simulink model "three_phase_hw_x"  (Simulink 6.1)
settings: Solver=ode23tb  StartTime=0.0  StopTime=0.14999  MaxStep=1e-4  RelTol=1e-3  AbsTol=.01
libraries: powerlib x17
settings Model: LastModifiedBy=ThinkPad
settings DebuggingCC: SolverPrmCheckMsg=warning

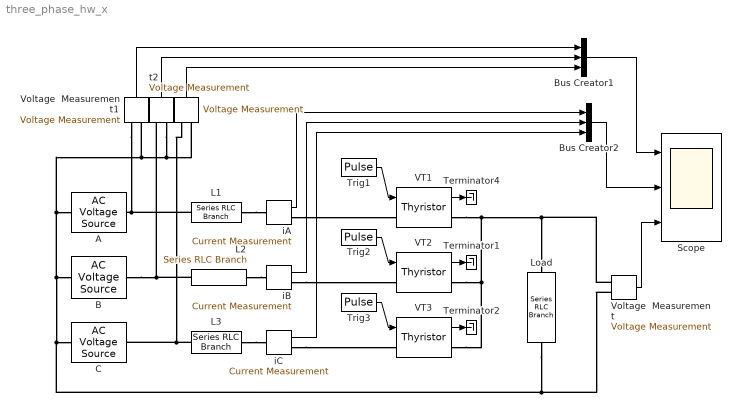
== system three_phase_hw_x ==
  "   " : powerlib/Measurements/Voltage Measurement  Orientation=up  PhasorSimulation=off  OutputType=Complex  PSBequivalent=0
  A : powerlib/Electrical Sources/AC Voltage Source  Amplitude=100  Phase=30  Frequency=50  SampleTime=0  Measurements=None
  B : powerlib/Electrical Sources/AC Voltage Source  Amplitude=100  Phase=-90  Frequency=50  SampleTime=0  Measurements=None
  Bus Creator1 : BusCreator  DialogController=Simulink.DDGSource_Bus  Inputs=3
  Bus Creator2 : BusCreator  DialogController=Simulink.DDGSource_Bus  Inputs=3
  C : powerlib/Electrical Sources/AC Voltage Source  Amplitude=100  Phase=-210  Frequency=50  SampleTime=0  Measurements=None
  L1 : powerlib/Elements/Series RLC Branch  Orientation=left  PhysicalDomain=powersysdomain  SubClassName=unknown  LeftPortType=p1  RightPortType=p1  LConnTagsString=__new0  RConnTagsString=__new0  Resistance=0  Inductance=0.002  Capacitance=inf  Measurements=None
  L2 : powerlib/Elements/Series RLC Branch  Orientation=left  PhysicalDomain=powersysdomain  SubClassName=unknown  LeftPortType=p1  RightPortType=p1  LConnTagsString=__new0  RConnTagsString=__new0  Resistance=0  Inductance=0.002  Capacitance=inf  Measurements=None
  L3 : powerlib/Elements/Series RLC Branch  Orientation=left  PhysicalDomain=powersysdomain  SubClassName=unknown  LeftPortType=p1  RightPortType=p1  LConnTagsString=__new0  RConnTagsString=__new0  Resistance=0  Inductance=0.002  Capacitance=inf  Measurements=None
  Load : powerlib/Elements/Series RLC Branch  Orientation=down  PhysicalDomain=powersysdomain  SubClassName=unknown  LeftPortType=p1  RightPortType=p1  LConnTagsString=__new0  RConnTagsString=__new0  Resistance=2  Inductance=0.05  Capacitance=inf  Measurements=None
  Scope : Scope  NumInputPorts=3
      settings: TimeRange=0.05  YMin=-100~0~-100  YMax=100~50~100  Decimation=5  SampleInput=on  SampleTime=1e-4
  Terminator1 : Terminator
  Terminator2 : Terminator
  Terminator4 : Terminator
  Trig1 : DiscretePulseGenerator  PulseType=Time based  Amplitude=10  Period=0.02  PulseWidth=5  PhaseDelay=0.00167
  Trig2 : DiscretePulseGenerator  PulseType=Time based  Amplitude=10  Period=0.02  PulseWidth=5  PhaseDelay=0.00833
  Trig3 : DiscretePulseGenerator  PulseType=Time based  Amplitude=10  Period=0.02  PulseWidth=5  PhaseDelay=0.015
  VT1 : powerlib/Power Electronics/Thyristor  Ron=0.01  Lon=0  Vf=0.8  IC=0  Rs=1000  Cs=100e-9  Measurements=on
  VT2 : powerlib/Power Electronics/Thyristor  Ron=0.01  Lon=0  Vf=0.8  IC=0  Rs=1000  Cs=100e-9  Measurements=on
  VT3 : powerlib/Power Electronics/Thyristor  Ron=0.01  Lon=0  Vf=0.8  IC=0  Rs=1000  Cs=100e-9  Measurements=on
  Voltage  Measurement : powerlib/Measurements/Voltage Measurement  PhasorSimulation=off  OutputType=Complex  PSBequivalent=0
  Voltage  Measurement1 : powerlib/Measurements/Voltage Measurement  Orientation=up  PhasorSimulation=off  OutputType=Complex  PSBequivalent=0
  iA : powerlib/Measurements/Current Measurement  PhasorSimulation=off  OutputType=Complex  PSBequivalent=0
  iB : powerlib/Measurements/Current Measurement  PhasorSimulation=off  OutputType=Complex  PSBequivalent=0
  iC : powerlib/Measurements/Current Measurement  PhasorSimulation=off  OutputType=Complex  PSBequivalent=0
  t2 : powerlib/Measurements/Voltage Measurement  Orientation=up  PhasorSimulation=off  OutputType=Complex  PSBequivalent=0
  wires:
  Voltage  Measurement/1 -> Scope/3
  Trig3/1 -> VT3/1
  Bus Creator1/1 -> Scope/1
  Voltage  Measurement1/1 -> Bus Creator1/1
  Trig2/1 -> VT2/1
  Bus Creator2/1 -> Scope/2
  Trig1/1 -> VT1/1
  t2/1 -> Bus Creator1/2
  "   "/1 -> Bus Creator1/3
  iA/1 -> Bus Creator2/1
  iB/1 -> Bus Creator2/2
  iC/1 -> Bus Creator2/3
  VT3/1 -> Terminator2/1
  VT2/1 -> Terminator1/1
  VT1/1 -> Terminator4/1
  connections:
  Voltage  Measurement/LConn2 -- B/LConn1 -- t2/LConn2 -- "   "/LConn2 -- Voltage  Measurement1/LConn2 -- A/LConn1 -- C/LConn1 -- Load/RConn1
  Voltage  Measurement1/LConn1 -- A/RConn1 -- L1/RConn1
  B/RConn1 -- t2/LConn1 -- L2/RConn1
  "   "/LConn1 -- C/RConn1 -- L3/RConn1
  Voltage  Measurement/LConn1 -- Load/LConn1 -- VT1/RConn1 -- VT3/RConn1 -- VT2/RConn1
  L1/LConn1 -- iA/LConn1
  iA/RConn1 -- VT1/LConn1
  L2/LConn1 -- iB/LConn1
  iB/RConn1 -- VT2/LConn1
  L3/LConn1 -- iC/LConn1
  iC/RConn1 -- VT3/LConn1
